simulink model "missile_model"  (R2022b)
settings: Solver=ode4  StartTime=0.0  StopTime=10.0  FixedStep=0.01  RelTol=1e-3
InitFcn:
  | clc, clear, close all
  | UAV_Data
  | Sim_Parameters
values from neighbouring files (symbols this model uses):
  Wn_Act = 25.0 * 2 * pi    (= 157.079632679)    [UAV_Data.m]    (also in UAV_Data.mat)
  Zeta_Act = 0.707    [UAV_Data.m]    (also in UAV_Data.mat)
settings Model: Creator=Komsun  LastModifiedBy=Komsun

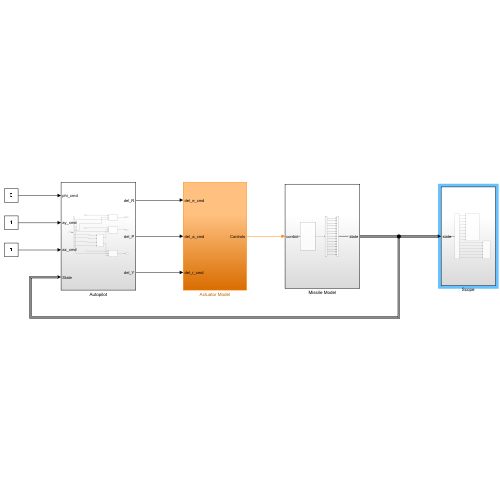
[thumbnail: Simulink's stored preview of the top-level diagram]
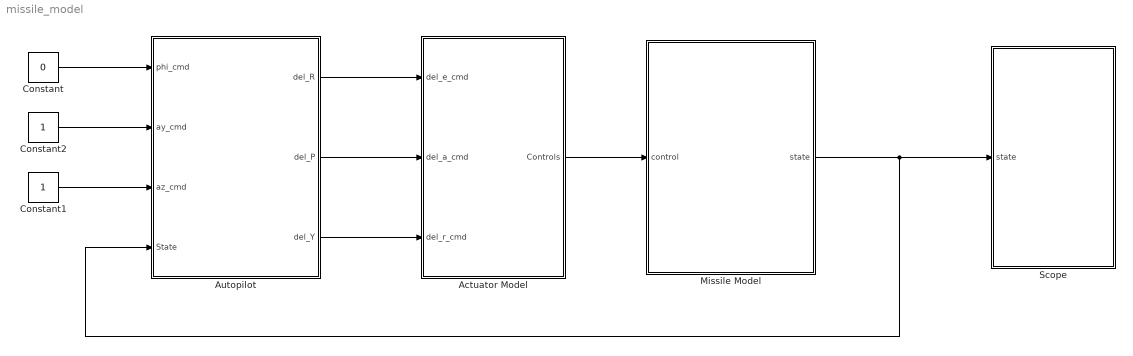
== system missile_model ==
  Actuator Model : Subsystem
  Autopilot : Subsystem
  Constant : Constant  Value=0
  Constant1 : Constant
  Constant2 : Constant
  Missile Model : Subsystem
  Scope : Subsystem
  wires:
  Constant2/1 -> Autopilot/2(ay_cmd)
  Constant1/1 -> Autopilot/3(az_cmd)
  Constant/1 -> Autopilot/1(phi_cmd)
  Missile Model/1(state) -> Autopilot/4(State), Scope/1(state)
  Actuator Model/1(Controls) -> Missile Model/1(control)
  Autopilot/1(del_R) -> Actuator Model/1(del_e_cmd)
  Autopilot/2(del_P) -> Actuator Model/2(del_a_cmd)
  Autopilot/3(del_Y) -> Actuator Model/3(del_r_cmd)

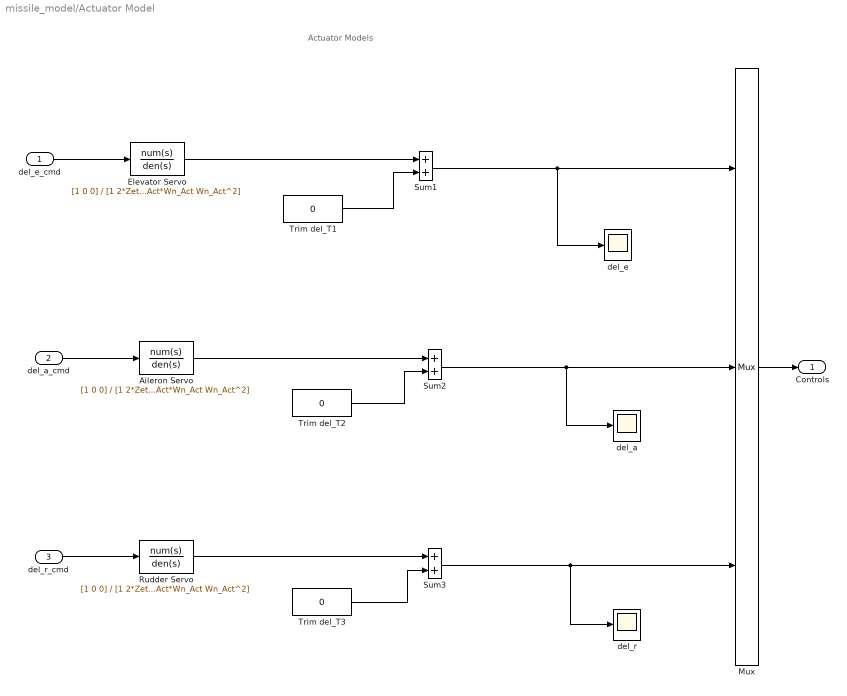
== system missile_model/Actuator Model ==
  note: Actuator Models
  del_e_cmd : Inport
  del_a_cmd : Inport  Port=2
  del_r_cmd : Inport  Port=3
  Aileron Servo : TransferFcn  Numerator=[1 0 0]  Denominator=[1 2*Zeta_Act*Wn_Act Wn_Act^2]
  Elevator Servo : TransferFcn  Numerator=[1 0 0]  Denominator=[1 2*Zeta_Act*Wn_Act Wn_Act^2]
  Mux : Mux  Inputs=3
  Rudder Servo : TransferFcn  Numerator=[1 0 0]  Denominator=[1 2*Zeta_Act*Wn_Act Wn_Act^2]
  Sum1 : Sum  SaturateOnIntegerOverflow=on
  Sum2 : Sum  SaturateOnIntegerOverflow=on
  Sum3 : Sum  SaturateOnIntegerOverflow=on
  Trim del_T1 : Constant  Value=0
  Trim del_T2 : Constant  Value=0
  Trim del_T3 : Constant  Value=0
  del_a : Scope
  del_e : Scope
  del_r : Scope
  Controls : Outport
  wires:
  Mux/1 -> Controls/1
  del_e_cmd/1 -> Elevator Servo/1
  Elevator Servo/1 -> Sum1/1
  Sum1/1 -> del_e/1, Mux/1
  Trim del_T1/1 -> Sum1/2
  Sum2/1 -> del_a/1, Mux/2
  Aileron Servo/1 -> Sum2/1
  Trim del_T2/1 -> Sum2/2
  del_a_cmd/1 -> Aileron Servo/1
  Sum3/1 -> Mux/3, del_r/1
  Trim del_T3/1 -> Sum3/2
  Rudder Servo/1 -> Sum3/1
  del_r_cmd/1 -> Rudder Servo/1

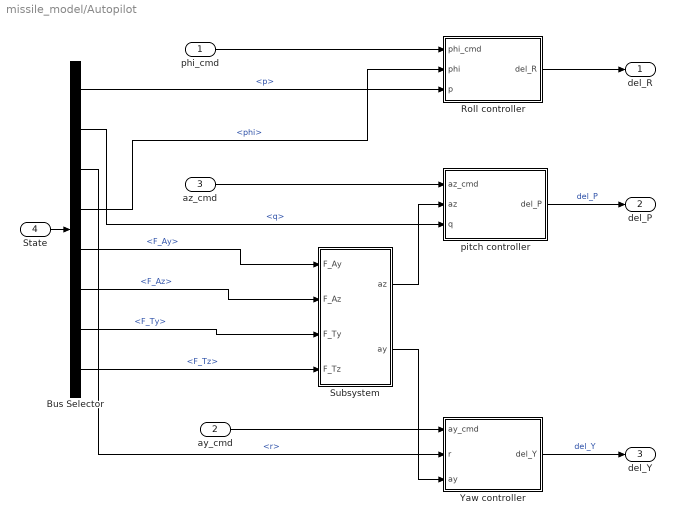
== system missile_model/Autopilot ==
  phi_cmd : Inport
  ay_cmd : Inport  Port=2
  az_cmd : Inport  Port=3
  State : Inport  Port=4
  Bus Selector : BusSelector  OutputSignals=p,q,r,phi,F_Ay,F_Az,F_Ty,F_Tz
  Roll controller : Subsystem
  Subsystem : Subsystem
  Yaw controller : Subsystem
  pitch controller : Subsystem
  del_R : Outport
  del_P : Outport  Port=2
  del_Y : Outport  Port=3
  wires:
  pitch controller/1(del_P) -> del_P/1  "del_P"
  Yaw controller/1(del_Y) -> del_Y/1  "del_Y"
  phi_cmd/1 -> Roll controller/1(phi_cmd)
  Roll controller/1(del_R) -> del_R/1
  az_cmd/1 -> pitch controller/1(az_cmd)
  Subsystem/1(az) -> pitch controller/2(az)
  ay_cmd/1 -> Yaw controller/1(ay_cmd)
  Subsystem/2(ay) -> Yaw controller/3(ay)
  State/1 -> Bus Selector/1
  Bus Selector/8 -> Subsystem/4(F_Tz)  "<F_Tz>"
  Bus Selector/7 -> Subsystem/3(F_Ty)  "<F_Ty>"
  Bus Selector/5 -> Subsystem/1(F_Ay)  "<F_Ay>"
  Bus Selector/6 -> Subsystem/2(F_Az)  "<F_Az>"
  Bus Selector/4 -> Roll controller/2(phi)  "<phi>"
  Bus Selector/3 -> Yaw controller/2(r)  "<r>"
  Bus Selector/2 -> pitch controller/3(q)  "<q>"
  Bus Selector/1 -> Roll controller/3(p)  "<p>"

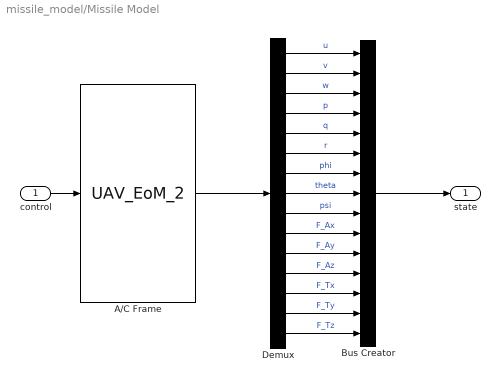
== system missile_model/Missile Model ==
  control : Inport
  A/C Frame : S-Function  FunctionName=UAV_EoM_2  SFunctionDeploymentMode=off  EnableBusSupport=off
  Bus Creator : BusCreator  Inputs=15
  Demux : Demux  Outputs=15
  state : Outport
  wires:
  control/1 -> A/C Frame/1
  Demux/14 -> Bus Creator/14  "F_Ty"
  A/C Frame/1 -> Demux/1
  Demux/6 -> Bus Creator/6  "r"
  Demux/13 -> Bus Creator/13  "F_Tx"
  Demux/10 -> Bus Creator/10  "F_Ax"
  Demux/3 -> Bus Creator/3  "w"
  Demux/4 -> Bus Creator/4  "p"
  Demux/5 -> Bus Creator/5  "q"
  Demux/2 -> Bus Creator/2  "v"
  Demux/1 -> Bus Creator/1  "u"
  Demux/9 -> Bus Creator/9  "psi"
  Demux/8 -> Bus Creator/8  "theta"
  Demux/11 -> Bus Creator/11  "F_Ay"
  Demux/7 -> Bus Creator/7  "phi"
  Demux/15 -> Bus Creator/15  "F_Tz"
  Demux/12 -> Bus Creator/12  "F_Az"
  Bus Creator/1 -> state/1

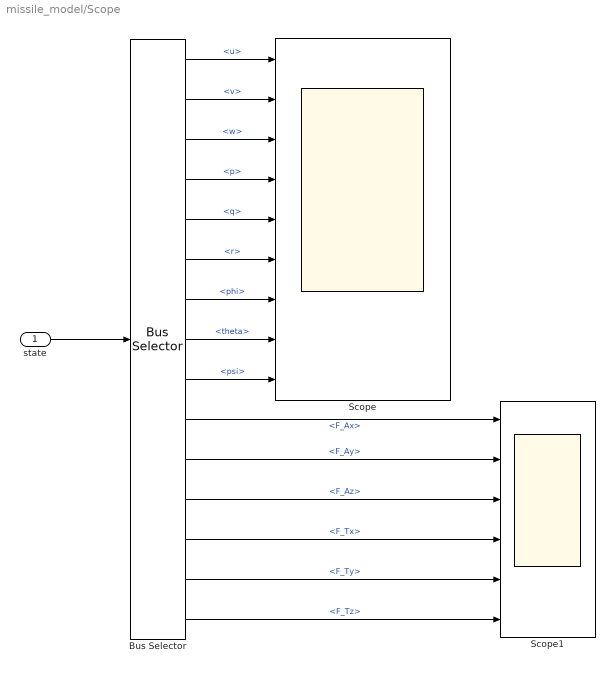
== system missile_model/Scope ==
  state : Inport
  Bus Selector : BusSelector  OutputSignals=u,v,w,p,q,r,phi,theta,psi,F_Ax,F_Ay,F_Az,F_Tx,F_Ty,F_Tz
  Scope : Scope  NumInputPorts=9
  Scope1 : Scope  NumInputPorts=6
  wires:
  state/1 -> Bus Selector/1
  Bus Selector/1 -> Scope/1  "<u>"
  Bus Selector/2 -> Scope/2  "<v>"
  Bus Selector/3 -> Scope/3  "<w>"
  Bus Selector/4 -> Scope/4  "<p>"
  Bus Selector/5 -> Scope/5  "<q>"
  Bus Selector/6 -> Scope/6  "<r>"
  Bus Selector/7 -> Scope/7  "<phi>"
  Bus Selector/8 -> Scope/8  "<theta>"
  Bus Selector/9 -> Scope/9  "<psi>"
  Bus Selector/10 -> Scope1/1  "<F_Ax>"
  Bus Selector/11 -> Scope1/2  "<F_Ay>"
  Bus Selector/12 -> Scope1/3  "<F_Az>"
  Bus Selector/13 -> Scope1/4  "<F_Tx>"
  Bus Selector/14 -> Scope1/5  "<F_Ty>"
  Bus Selector/15 -> Scope1/6  "<F_Tz>"

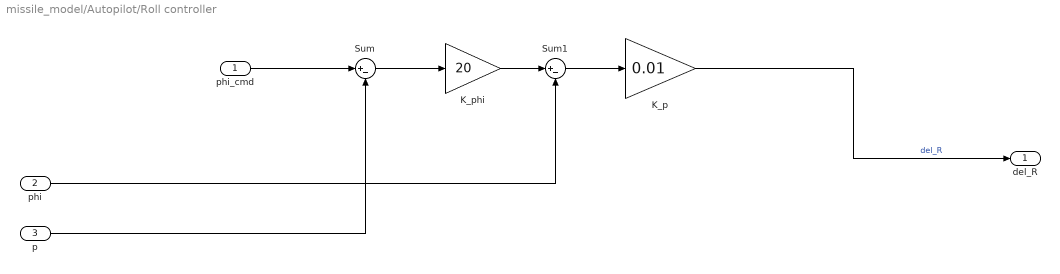
== system missile_model/Autopilot/Roll controller ==
  phi_cmd : Inport
  phi : Inport  Port=2
  p : Inport  Port=3
  K_p : Gain  Gain=0.01
  K_phi : Gain  Gain=20
  Sum : Sum  Inputs=|+-
  Sum1 : Sum  Inputs=|+-
  del_R : Outport
  wires:
  p/1 -> Sum/2
  K_p/1 -> del_R/1  "del_R"
  Sum/1 -> K_phi/1
  phi/1 -> Sum1/2
  Sum1/1 -> K_p/1
  K_phi/1 -> Sum1/1
  phi_cmd/1 -> Sum/1

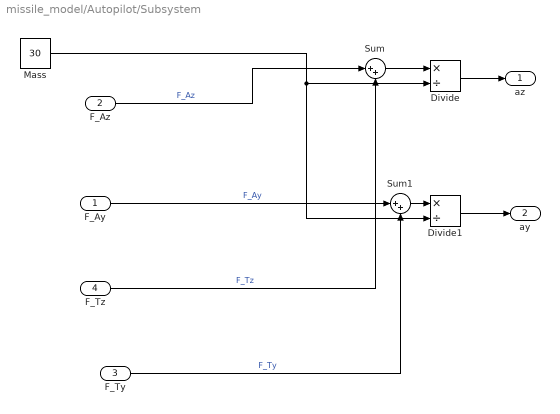
== system missile_model/Autopilot/Subsystem ==
  F_Ay : Inport
  F_Az : Inport  Port=2
  F_Ty : Inport  Port=3
  F_Tz : Inport  Port=4
  Divide : Product  Inputs=*/
  Divide1 : Product  Inputs=*/
  Mass : Constant  Value=30
  Sum : Sum  Inputs=|++
  Sum1 : Sum  Inputs=|++
  az : Outport
  ay : Outport  Port=2
  wires:
  F_Ay/1 -> Sum1/1  "F_Ay"
  Mass/1 -> Divide1/2, Divide/2
  Sum/1 -> Divide/1
  F_Ty/1 -> Sum1/2  "F_Ty"
  Sum1/1 -> Divide1/1
  F_Az/1 -> Sum/1  "F_Az"
  Divide/1 -> az/1
  F_Tz/1 -> Sum/2  "F_Tz"
  Divide1/1 -> ay/1

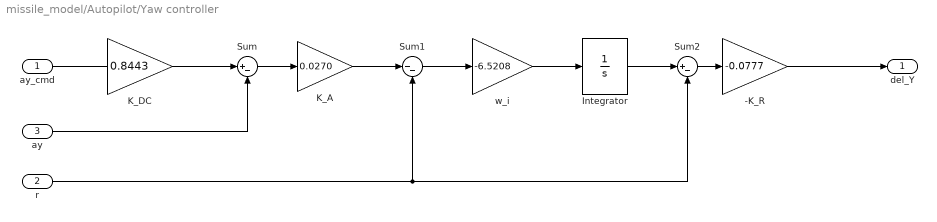
== system missile_model/Autopilot/Yaw controller ==
  ay_cmd : Inport
  r : Inport  Port=2
  ay : Inport  Port=3
  -K_R : Gain  Gain=-0.0777
  Integrator : Integrator
  K_A : Gain  Gain=0.0270
  K_DC : Gain  Gain=0.8443
  Sum : Sum  Inputs=|+-
  Sum1 : Sum  Inputs=|--
  Sum2 : Sum  Inputs=|+-
  w_i : Gain  Gain=-6.5208
  del_Y : Outport
  wires:
  ay_cmd/1 -> ?
  r/1 -> Sum2/2, Sum1/2
  K_DC/1 -> Sum/1
  ay/1 -> Sum/2
  Sum/1 -> K_A/1
  K_A/1 -> Sum1/1
  Sum1/1 -> w_i/1
  w_i/1 -> Integrator/1
  Integrator/1 -> Sum2/1
  Sum2/1 -> -K_R/1
  -K_R/1 -> del_Y/1

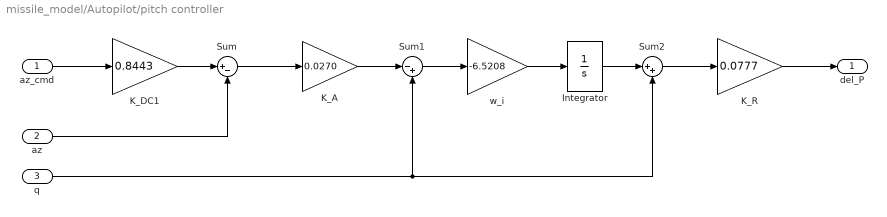
== system missile_model/Autopilot/pitch controller ==
  az_cmd : Inport
  az : Inport  Port=2
  q : Inport  Port=3
  Integrator : Integrator
  K_A : Gain  Gain=0.0270
  K_DC1 : Gain  Gain=0.8443
  K_R : Gain  Gain=0.0777
  Sum : Sum  Inputs=|+-
  Sum1 : Sum  Inputs=|-+
  Sum2 : Sum  Inputs=|++
  w_i : Gain  Gain=-6.5208
  del_P : Outport
  wires:
  az_cmd/1 -> K_DC1/1
  K_DC1/1 -> Sum/1
  az/1 -> Sum/2
  Sum/1 -> K_A/1
  K_A/1 -> Sum1/1
  q/1 -> Sum2/2, Sum1/2
  Sum1/1 -> w_i/1
  w_i/1 -> Integrator/1
  Integrator/1 -> Sum2/1
  Sum2/1 -> K_R/1
  K_R/1 -> del_P/1
